simulink library "lib_Servo"  (R2018b)
settings: Solver=VariableStepAuto  StartTime=0.0  StopTime=10.0  RelTol=1e-3
undefined symbols (not defined in the file): FCC_PIX_Data, HIL_Data
libraries: $bdroot x9
settings Model: Creator=m.hiepp  LastModifiedBy=m.hiepp

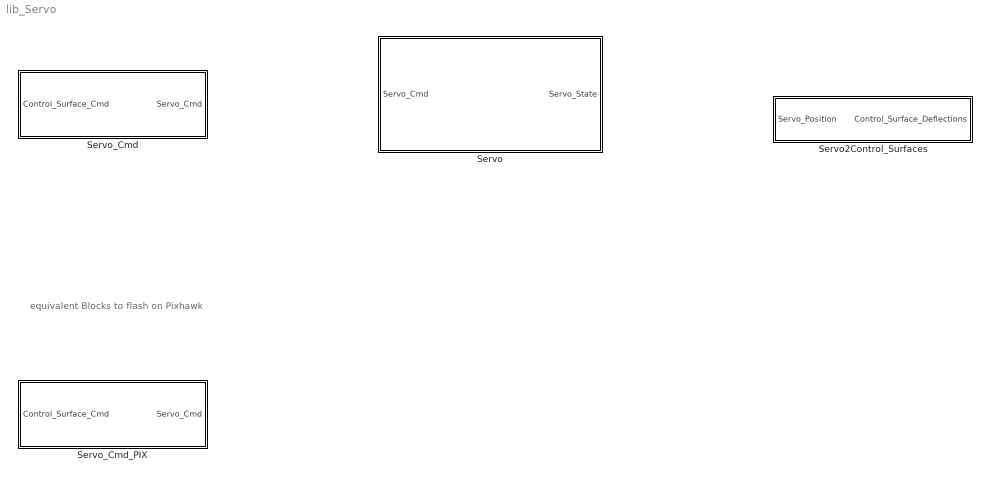
== system lib_Servo ==
  note: equivalent Blocks to flash on Pixhawk
  Servo : Subsystem  mask{TF=HIL_Data.Servo.TF, PWM=HIL_Data.Servo.PWM}
      mask prompts: TF "Transer Function"; PWM "PWM Data"
  Servo2Control_Surfaces : Subsystem
  Servo_Cmd : Subsystem  mask{PWM=HIL_Data.Servo.PWM, Control_Surfaces=HIL_Data.Control_Surfaces}
      mask prompts: PWM "PWM Data"; Control_Surfaces "Control Surfaces Data"
  Servo_Cmd_PIX : Subsystem

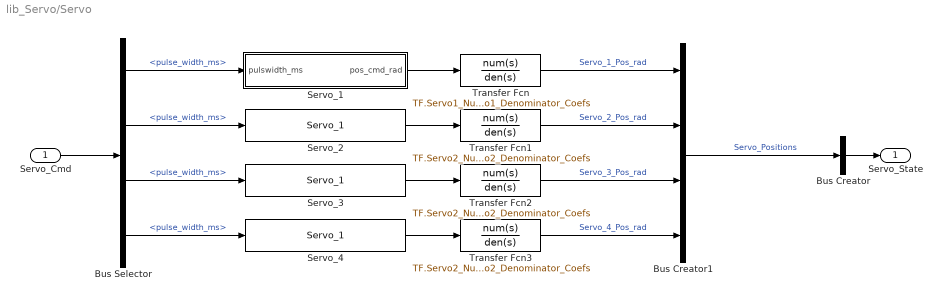
== system lib_Servo/Servo ==
  Servo_Cmd : Inport  OutDataTypeStr=Bus: Servo_Cmd_Bus
  Bus Creator : BusCreator  Inputs=1  OutDataTypeStr=Bus: Servo_State_Bus
  Bus Creator1 : BusCreator  Inputs=4  OutDataTypeStr=Bus: Servo_Positions_Bus
  Bus Selector : BusSelector  OutputSignals=Servo_1_Cmd_PWM.pulse_width_ms,Servo_2_Cmd_PWM.pulse_width_ms,Servo_3_Cmd_PWM.pulse_width_ms,Servo_4_Cmd_PWM.pulse_width_ms
  Servo_1 : Subsystem
  Servo_2 : $bdroot/Servo/Servo_1  SystemSampleTime=-1
  Servo_3 : $bdroot/Servo/Servo_1  SystemSampleTime=-1
  Servo_4 : $bdroot/Servo/Servo_1  SystemSampleTime=-1
  Transfer Fcn : TransferFcn  Numerator=TF.Servo1_Numerator_Coefs  Denominator=TF.Servo1_Denominator_Coefs
  Transfer Fcn1 : TransferFcn  Numerator=TF.Servo2_Numerator_Coefs  Denominator=TF.Servo2_Denominator_Coefs
  Transfer Fcn2 : TransferFcn  Numerator=TF.Servo2_Numerator_Coefs  Denominator=TF.Servo2_Denominator_Coefs
  Transfer Fcn3 : TransferFcn  Numerator=TF.Servo2_Numerator_Coefs  Denominator=TF.Servo2_Denominator_Coefs
  Servo_State : Outport  OutDataTypeStr=Bus: Servo_State_Bus
  wires:
  Servo_Cmd/1 -> Bus Selector/1
  Bus Creator/1 -> Servo_State/1
  Bus Creator1/1 -> Bus Creator/1  "Servo_Positions"
  Transfer Fcn/1 -> Bus Creator1/1  "Servo_1_Pos_rad"
  Transfer Fcn1/1 -> Bus Creator1/2  "Servo_2_Pos_rad"
  Transfer Fcn2/1 -> Bus Creator1/3  "Servo_3_Pos_rad"
  Transfer Fcn3/1 -> Bus Creator1/4  "Servo_4_Pos_rad"
  Servo_1/1(pos_cmd_rad) -> Transfer Fcn/1
  Bus Selector/1 -> Servo_1/1(pulswidth_ms)  "<pulse_width_ms>"
  Servo_4/1 -> Transfer Fcn3/1
  Bus Selector/4 -> Servo_4/1  "<pulse_width_ms>"
  Servo_3/1 -> Transfer Fcn2/1
  Bus Selector/3 -> Servo_3/1  "<pulse_width_ms>"
  Servo_2/1 -> Transfer Fcn1/1
  Bus Selector/2 -> Servo_2/1  "<pulse_width_ms>"

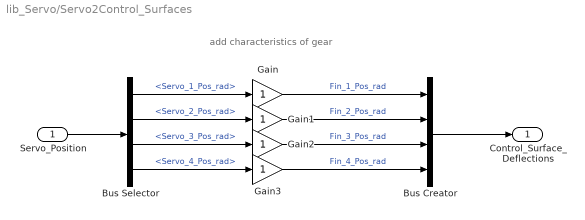
== system lib_Servo/Servo2Control_Surfaces ==
  note: add characteristics of gear
  Servo_Position : Inport  OutDataTypeStr=Bus: Servo_Positions_Bus
  Bus Creator : BusCreator  Inputs=4  OutDataTypeStr=Bus: Control_Surface_Deflections_Bus
  Bus Selector : BusSelector  OutputSignals=Servo_1_Pos_rad,Servo_2_Pos_rad,Servo_3_Pos_rad,Servo_4_Pos_rad
  Gain{,1..3} (4 alike) : Gain
  Control_Surface_Deflections : Outport  OutDataTypeStr=Bus: Control_Surface_Deflections_Bus
  wires:
  Servo_Position/1 -> Bus Selector/1
  Bus Creator/1 -> Control_Surface_Deflections/1
  Bus Selector/1 -> Gain/1  "<Servo_1_Pos_rad>"
  Bus Selector/2 -> Gain1/1  "<Servo_2_Pos_rad>"
  Bus Selector/3 -> Gain2/1  "<Servo_3_Pos_rad>"
  Bus Selector/4 -> Gain3/1  "<Servo_4_Pos_rad>"
  Gain/1 -> Bus Creator/1  "Fin_1_Pos_rad"
  Gain1/1 -> Bus Creator/2  "Fin_2_Pos_rad"
  Gain2/1 -> Bus Creator/3  "Fin_3_Pos_rad"
  Gain3/1 -> Bus Creator/4  "Fin_4_Pos_rad"

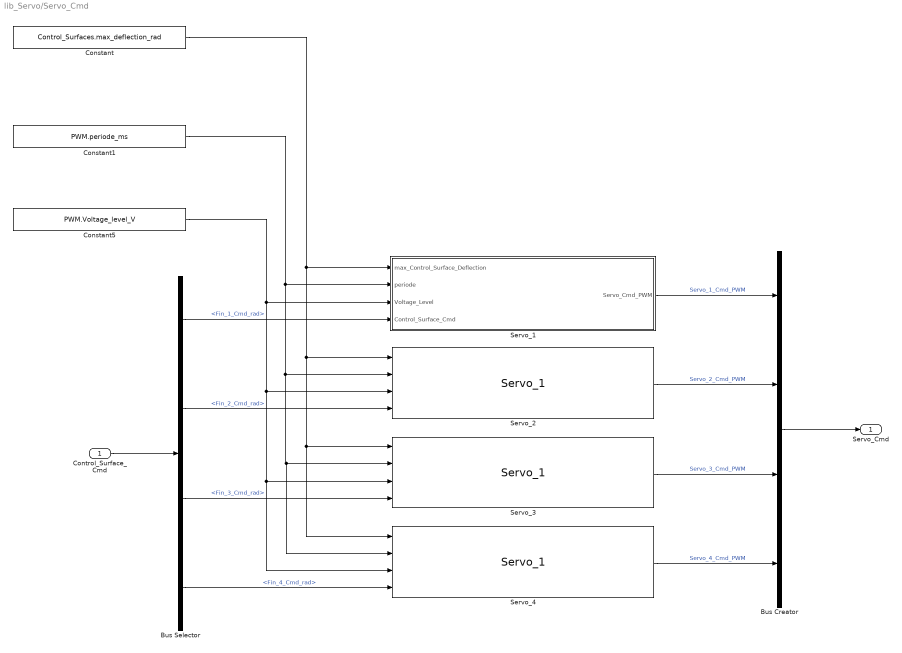
== system lib_Servo/Servo_Cmd ==
  Control_Surface_Cmd : Inport  OutDataTypeStr=Bus: Control_Surface_Cmd_Bus
  Bus Creator : BusCreator  Inputs=4  OutDataTypeStr=Bus: Servo_Cmd_Bus
  Bus Selector : BusSelector  OutputSignals=Fin_1_Cmd_rad,Fin_2_Cmd_rad,Fin_3_Cmd_rad,Fin_4_Cmd_rad
  Constant : Constant  Value=Control_Surfaces.max_deflection_rad
  Constant1 : Constant  Value=PWM.periode_ms
  Constant5 : Constant  Value=PWM.Voltage_level_V
  Servo_1 : Subsystem
  Servo_2 : $bdroot/Servo_Cmd/Servo_1  SystemSampleTime=-1
  Servo_3 : $bdroot/Servo_Cmd/Servo_1  SystemSampleTime=-1
  Servo_4 : $bdroot/Servo_Cmd/Servo_1  SystemSampleTime=-1
  Servo_Cmd : Outport  OutDataTypeStr=Bus: Servo_Cmd_Bus
  wires:
  Control_Surface_Cmd/1 -> Bus Selector/1
  Bus Creator/1 -> Servo_Cmd/1
  Servo_1/1(Servo_Cmd_PWM) -> Bus Creator/1  "Servo_1_Cmd_PWM"
  Constant/1 -> Servo_4/1, Servo_3/1, Servo_2/1, Servo_1/1(max_Control_Surface_Deflection)
  Constant1/1 -> Servo_4/2, Servo_3/2, Servo_2/2, Servo_1/2(periode)
  Constant5/1 -> Servo_2/3, Servo_4/3, Servo_3/3, Servo_1/3(Voltage_Level)
  Servo_2/1 -> Bus Creator/2  "Servo_2_Cmd_PWM"
  Servo_3/1 -> Bus Creator/3  "Servo_3_Cmd_PWM"
  Servo_4/1 -> Bus Creator/4  "Servo_4_Cmd_PWM"
  Bus Selector/4 -> Servo_4/4  "<Fin_4_Cmd_rad>"
  Bus Selector/3 -> Servo_3/4  "<Fin_3_Cmd_rad>"
  Bus Selector/2 -> Servo_2/4  "<Fin_2_Cmd_rad>"
  Bus Selector/1 -> Servo_1/4(Control_Surface_Cmd)  "<Fin_1_Cmd_rad>"

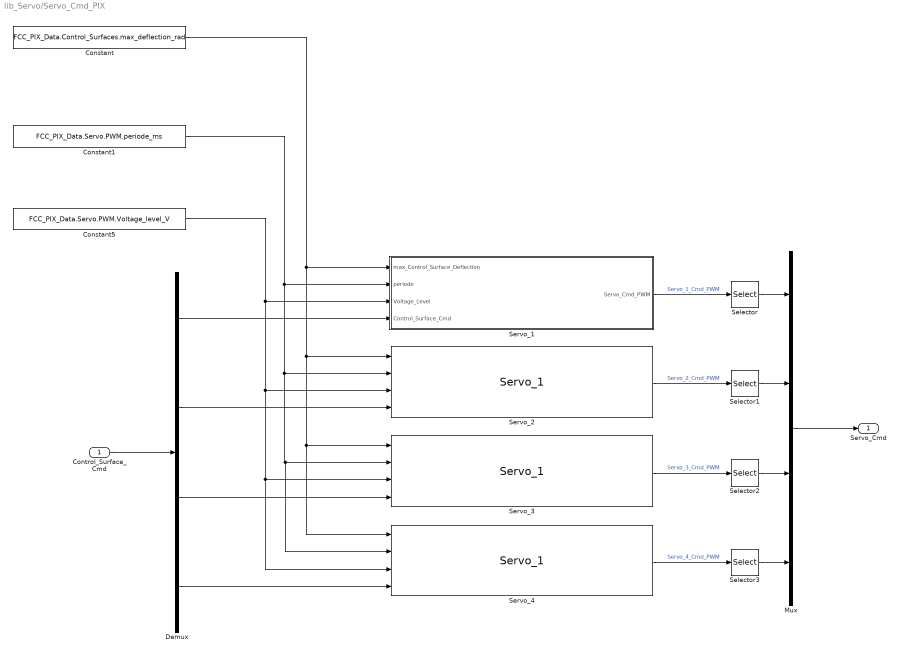
== system lib_Servo/Servo_Cmd_PIX ==
  Control_Surface_Cmd : Inport
  Constant : Constant  Value=FCC_PIX_Data.Control_Surfaces.max_deflection_rad
  Constant1 : Constant  Value=FCC_PIX_Data.Servo.PWM.periode_ms
  Constant5 : Constant  Value=FCC_PIX_Data.Servo.PWM.Voltage_level_V
  Demux : Demux
  Mux : Mux
  Selector{,1..3} (4 alike) : Selector  InputPortWidth=3  IndexOptions=Index vector (dialog)  Indices=[1]  OutputSizes=1
  Servo_1 : Subsystem
  Servo_2 : $bdroot/Servo_Cmd_PIX/Servo_1  SystemSampleTime=-1
  Servo_3 : $bdroot/Servo_Cmd_PIX/Servo_1  SystemSampleTime=-1
  Servo_4 : $bdroot/Servo_Cmd_PIX/Servo_1  SystemSampleTime=-1
  Servo_Cmd : Outport
  wires:
  Control_Surface_Cmd/1 -> Demux/1
  Mux/1 -> Servo_Cmd/1
  Servo_1/1(Servo_Cmd_PWM) -> Selector/1  "Servo_1_Cmd_PWM"
  Constant/1 -> Servo_2/1, Servo_4/1, Servo_3/1, Servo_1/1(max_Control_Surface_Deflection)
  Constant1/1 -> Servo_2/2, Servo_4/2, Servo_3/2, Servo_1/2(periode)
  Constant5/1 -> Servo_2/3, Servo_4/3, Servo_3/3, Servo_1/3(Voltage_Level)
  Servo_2/1 -> Selector1/1  "Servo_2_Cmd_PWM"
  Servo_3/1 -> Selector2/1  "Servo_3_Cmd_PWM"
  Servo_4/1 -> Selector3/1  "Servo_4_Cmd_PWM"
  Demux/4 -> Servo_4/4
  Demux/3 -> Servo_3/4
  Demux/2 -> Servo_2/4
  Demux/1 -> Servo_1/4(Control_Surface_Cmd)
  Selector1/1 -> Mux/2
  Selector/1 -> Mux/1
  Selector2/1 -> Mux/3
  Selector3/1 -> Mux/4

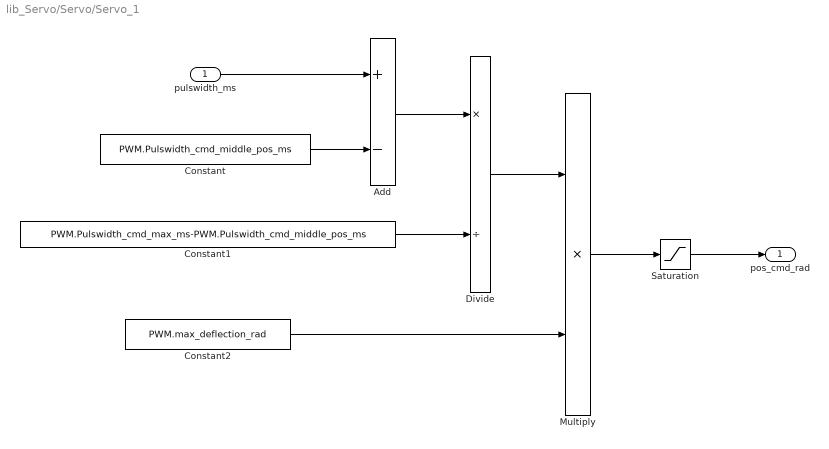
== system lib_Servo/Servo/Servo_1 ==
  pulswidth_ms : Inport
  Add : Sum  Inputs=+-
  Constant : Constant  Value=PWM.Pulswidth_cmd_middle_pos_ms
  Constant1 : Constant  Value=PWM.Pulswidth_cmd_max_ms-PWM.Pulswidth_cmd_middle_pos_ms
  Constant2 : Constant  Value=PWM.max_deflection_rad
  Divide : Product  Inputs=*/
  Multiply : Product
  Saturation : Saturate  UpperLimit=PWM.max_deflection_rad  LowerLimit=-PWM.max_deflection_rad
  pos_cmd_rad : Outport
  wires:
  Constant/1 -> Add/2
  pulswidth_ms/1 -> Add/1
  Add/1 -> Divide/1
  Constant1/1 -> Divide/2
  Divide/1 -> Multiply/1
  Constant2/1 -> Multiply/2
  Multiply/1 -> Saturation/1
  Saturation/1 -> pos_cmd_rad/1

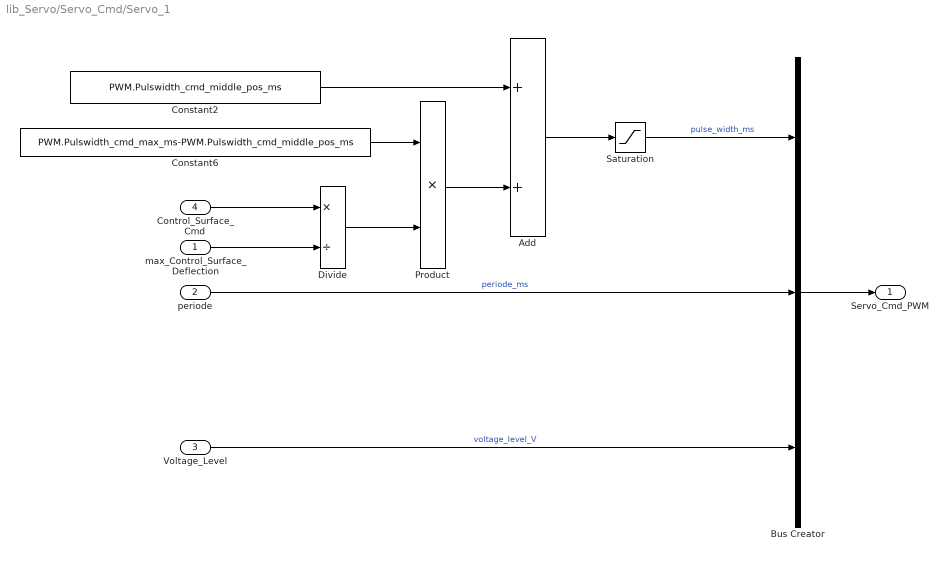
== system lib_Servo/Servo_Cmd/Servo_1 ==
  max_Control_Surface_Deflection : Inport
  periode : Inport  Port=2
  Voltage_Level : Inport  Port=3
  Control_Surface_Cmd : Inport  Port=4
  Add : Sum
  Bus Creator : BusCreator  Inputs=3  OutDataTypeStr=Bus: PWM_Cmd_Bus
  Constant2 : Constant  Value=PWM.Pulswidth_cmd_middle_pos_ms
  Constant6 : Constant  Value=PWM.Pulswidth_cmd_max_ms-PWM.Pulswidth_cmd_middle_pos_ms
  Divide : Product  Inputs=*/
  Product : Product
  Saturation : Saturate  UpperLimit=PWM.Pulswidth_cmd_max_ms  LowerLimit=PWM.Pulswidth_cmd_min_ms
  Servo_Cmd_PWM : Outport
  wires:
  Constant2/1 -> Add/1
  Divide/1 -> Product/2
  Add/1 -> Saturation/1
  Voltage_Level/1 -> Bus Creator/3  "voltage_level_V"
  Control_Surface_Cmd/1 -> Divide/1
  Product/1 -> Add/2
  Constant6/1 -> Product/1
  Saturation/1 -> Bus Creator/1  "pulse_width_ms"
  periode/1 -> Bus Creator/2  "periode_ms"
  max_Control_Surface_Deflection/1 -> Divide/2
  Bus Creator/1 -> Servo_Cmd_PWM/1

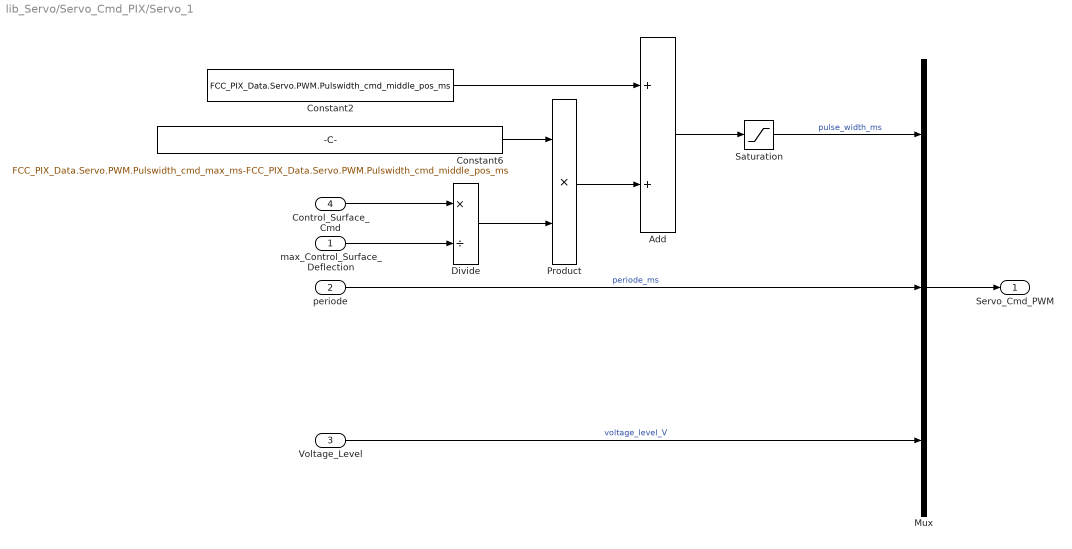
== system lib_Servo/Servo_Cmd_PIX/Servo_1 ==
  max_Control_Surface_Deflection : Inport
  periode : Inport  Port=2
  Voltage_Level : Inport  Port=3
  Control_Surface_Cmd : Inport  Port=4
  Add : Sum
  Constant2 : Constant  Value=FCC_PIX_Data.Servo.PWM.Pulswidth_cmd_middle_pos_ms
  Constant6 : Constant  Value=FCC_PIX_Data.Servo.PWM.Pulswidth_cmd_max_ms-FCC_PIX_Data.Servo.PWM.Pulswidth_cmd_middle_pos_ms
  Divide : Product  Inputs=*/
  Mux : Mux  Inputs=3
  Product : Product
  Saturation : Saturate  UpperLimit=FCC_PIX_Data.Servo.PWM.Pulswidth_cmd_max_ms  LowerLimit=FCC_PIX_Data.Servo.PWM.Pulswidth_cmd_min_ms
  Servo_Cmd_PWM : Outport
  wires:
  Constant2/1 -> Add/1
  Divide/1 -> Product/2
  Add/1 -> Saturation/1
  Voltage_Level/1 -> Mux/3  "voltage_level_V"
  Control_Surface_Cmd/1 -> Divide/1
  Product/1 -> Add/2
  Constant6/1 -> Product/1
  Saturation/1 -> Mux/1  "pulse_width_ms"
  periode/1 -> Mux/2  "periode_ms"
  max_Control_Surface_Deflection/1 -> Divide/2
  Mux/1 -> Servo_Cmd_PWM/1
